simulink model "Plant"  (R2021a)
settings: Solver=VariableStepAuto  StartTime=0.0  StopTime=10.0  RelTol=1e-3
values from neighbouring files (symbols this model uses):
  bcx = 1e7    (= 10000000)    [Data.m]
  bcy = 1e8    (= 100000000)    [Data.m]
  bEh = 2*(bhd + bhm*ih^2)/rhd^2    (= 31004.4444444)    [Data.m]
  bEtd = (btd + btm*it^2)/rtd^2    (= 21607.2)    [Data.m]
  bhb = 1.0e8    (= 100000000)    [Data.m]
  bhEb = 2.2e9    (= 2200000000)    [Data.m]
  bt = 90    [Data.m]
  btb = 5.0e6    (= 5000000)    [Data.m]
  btw = 3e3    (= 3000)    [Data.m]
  bwu = 150    [Data.m]
  Container1_x0 = -15    [Data.m]
  Container1_y0 = 2.2    [Data.m]
  containerLayout = randi([0, maxContainers], 1, columns)    [Data.m]
  containerMasses = randi([Mc_range(1), Mc_range(2)], 1, columns)    [Data.m]
  dlh0 = 0    [Data.m]    (also in test__TLK.m; test_hoist.m; test_trolley.m)
  dxt0 = 0    [Data.m]    (also in test__TLK.m; test_hoist.m; test_trolley.m)
  dxtd0 = 0    [Data.m]    (also in test__TLK.m; test_hoist.m; test_trolley.m)
  g = 9.80665    [Data.m]
  Hc = 2.5    [Data.m]
  hoist_v115 = 115    [Data.m]
  ih = 22    [Data.m]
  it = 30    [Data.m]
  Kcy = 1.8e9    (= 1800000000)    [Data.m]
  Ktw = 4.8e5    (= 480000)    [Data.m]
  kwu = 2.36e8    (= 236000000)    [Data.m]
  lh0 = 10    [Data.m]    (also in test__TLK.m = 54.35; test_hoist.m = 20; test_trolley.m = 6)
  MAX_CABLE_LENGTH = y_axis(2) - y_axis(1)    [Data.m]
  Mc_range = [2000 50000]    [Data.m]
  MEh = 2*(Jhd_hEb + Jhm_hb * ih^2)/rhd^2    (= 65137.7777778)    [Data.m]
  MEtd = (Jtd + Jtm_tb*it^2)/rtd^2    (= 30000)    [Data.m]
  Ms = 15000    [Data.m]
  Mt = 30000    [Data.m]
  rhd = 0.75    [Data.m]
  rtd = 0.5    [Data.m]
  SHIP_LIMIT = x_axis(2)    [Data.m]
  SHORE_LIMIT = x_axis(1)    [Data.m]
  Thb_max = 5.0e4    (= 50000)    [Data.m]
  ThEb_max = 1.1e6    (= 1100000)    [Data.m]
  theta_hm0 = 0    [Data.m]    (also in test__TLK.m; test_hoist.m; test_trolley.m)
  theta_tm0 = 0    [Data.m]    (also in test__TLK.m; test_hoist.m; test_trolley.m)
  Ttb_max = 5.0e-3    (= 0.005)    [Data.m]
  Vlx0 = 0    [Data.m]    (also in test__TLK.m; test_hoist.m; test_trolley.m)
  Vly0 = 0    [Data.m]    (also in test__TLK.m; test_hoist.m; test_trolley.m)
  x_axis = [-30 50]    [Data.m]
  xl0 = xt0    (= 1)    [Data.m]    (also in test__TLK.m = 10.55; test_hoist.m = -20; test_trolley.m = -25)
  xt0 = 1    [Data.m]    (also in test__TLK.m = 10.55; test_hoist.m = -20; test_trolley.m = -25)
  xtd0 = xt0    (= 1)    [Data.m]    (also in test__TLK.m = 10.55; test_hoist.m = -20; test_trolley.m = -25)
  y_axis = [-20 40]    [Data.m]
  yl0 = Yt0 - lh0    (= 35)    [Data.m]    (also in test__TLK.m = Yt0 - lh0; test_hoist.m = Yt0 - lh0; test_trolley.m = Yt0 - lh0 - 1/4 * (Ms*g)/(kwu/(2*lh0+110)))
  Yt0 = 45    [Data.m]
libraries: simulink x3, vrlib x1
settings Model: Creator=jpss8  LastModifiedBy=ThnkPad

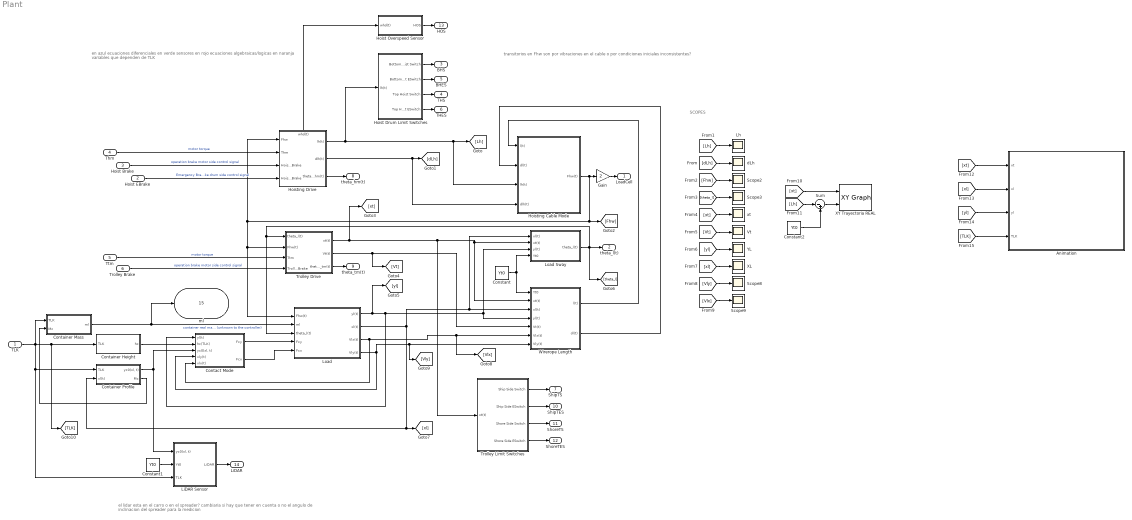
== system Plant ==
  note: SCOPES
  note: en azul ecuaciones diferenciales
      | en verde sensores
      | en rojo ecuaciones algebraicas/logicas
      | en naranja variables que dependen de TLK
  note: el lidar esta en el carro o en el spreader? cambiaria si hay que tener en cuenta o no el angulo de inclinacion del spreader para la medicion
  note: transitorios en Fhw son por vibraciones en el cable o por condiciones iniciales inconsistentes?
  TLK : Inport
  Hoist EBrake : Inport  Port=2
  Hoist Brake : Inport  Port=3
  Thm : Inport  Port=4
  Ttm : Inport  Port=5
  Trolley Brake : Inport  Port=6
  Animation : Subsystem
  Constant : Constant  Value=Yt0
  Constant1 : Constant  Value=Yt0
  Constant2 : Constant  Value=Yt0
  Contact Mode : Subsystem
  Container Height : Subsystem
  Container Mass : Subsystem
  Container Profile : Subsystem
  Gain : Gain  Gain=2
  Hoist Drum Limit Switches : Subsystem
  Hoist Overspeed Sensor : Subsystem
  Hoisting Cable Mode : Subsystem
  Hoisting Drive : Subsystem
      settings: PortSchema="{\"entries\":[{\"content\":{\"sides\":[{\"content\":{\"connectorIds\":[\"In1\",\"In2\",\"In3\",\"In4\"]},\"type\":\"ConnectorPlacement.EquallySpacedRectSide\",\"uuid\":\"6fd1770e-d7ed-4f51-91a0-0929c8efe1d3\"},{\"content\":{\"connectorIds\":[\"Out1\",\"Out2\",\"Out3\"],\"side\":\"RIGHT\"},\"type\":\"ConnectorPlacement.EquallySpacedRectSide\",\"uuid\":\"8b4207e8-a8fb-49cf-b187-d50d58bbe698\"},{\"content\":{\"connectorIds\":[\"Out4\"],\"side\":\"TOP\"},\"type\":\"ConnectorPlacement.EquallySpacedRectSide\",\"uuid\":\"5319a049-552f-4b27-a7d1-196eaf1861ff\"}]},\"type\":\"ConnectorPlacement.EquallySpacedConnector\",\"uuid\":\"15d51aa7-7d1b-46b1-a1b4-72147bb9bc95\"}],\"packageUris\":[\"http://schema.mathworks.com/mf0/Connector/R2020b\"],\"version\":\"1.0\"}"
  Lh : Scope
  LiDAR Sensor : Subsystem
  Load : Subsystem
  Load Sway : Subsystem
  Scope{2..3,8..9} (4 alike) : Scope
  Sum : Sum  Inputs=|-+
  Trolley Drive : Subsystem
  Trolley Limit Switches : Subsystem
  Vt : Scope
  Wirerope Length : Subsystem
  XL : Scope
  XY Trayectoria REAL : simulink/Sinks/XY Graph  xmin=x_axis(1)  xmax=x_axis(2)  ymin=y_axis(1)  ymax=y_axis(2)  st=-1
  YL : Scope
  dLh : Scope
  xt : Scope
  LoadCell : Outport
  theta_l(t) : Outport  Port=2
  BHS : Outport  Port=3
  THS : Outport  Port=4
  BHES : Outport  Port=5
  THES : Outport  Port=6
  ShipTS : Outport  Port=7
  theta_hm(t) : Outport  Port=8
  theta_tm(t) : Outport  Port=9
  ShipTES : Outport  Port=10
  ShoreTS : Outport  Port=11
  ShoreTES : Outport  Port=12
  HOS : Outport  Port=13
  LiDAR : Outport  Port=14
  ml : Outport  Port=15
  wires:
  Load/2(xl(t)) -> [xl], Container Profile/2(xl(t)), Load Sway/1(xl(t)), Wirerope Length/3(xl(t))
  Constant/1 -> Load Sway/4(Yt0), Wirerope Length/1(Yt0)
  Contact Mode/1(Fcy) -> Load/4(Fcy)
  Contact Mode/2(Fcx) -> Load/5(Fcx)
  Load/4(Vly(t)) -> Contact Mode/4(vly(t)), [Vly], Wirerope Length/7(Vly(t))
  Load/3(Vlx(t)) -> Contact Mode/5(vlx(t)), [Vlx], Wirerope Length/6(Vlx(t))
  Container Height/1(hc) -> Contact Mode/2(hc(TLK))
  Load Sway/1(theta_l(t)) -> [theta_l], theta_l(t)/1, Load/3(theta_l(t)), Trolley Drive/1(theta_l(t))
  Container Mass/1(ml) -> ml/1, Load/2(ml)  "container real mass (unknown to the controller)"
  Trolley Drive/1(xt(t)) -> [xt], Trolley Limit Switches/1(xt(t)), Wirerope Length/2(xt(t)), Load Sway/2(xt(t))
  Hoisting Drive/1(lh(t)) -> Hoist Drum Limit Switches/1(lh(t)), [Lh], Hoisting Cable Mode/3(lh(t))
  Hoisting Drive/2(dlh(t)) -> Hoisting Cable Mode/4(dlh(t)), [dLh]
  Wirerope Length/1(l(t)) -> Hoisting Cable Mode/1(l(t))
  Wirerope Length/2(dl(t)) -> Hoisting Cable Mode/2(dl(t))
  Hoisting Cable Mode/1(Fhw(t)) -> Gain/1, [Fhw], Load/1(Fhw(t)), Trolley Drive/2(Fhw(t)), Hoisting Drive/1(Fhw)
  Ttm/1 -> Trolley Drive/3(Ttm)  "motor torque"
  Thm/1 -> Hoisting Drive/2(Thm)  "motor torque"
  Trolley Brake/1 -> Trolley Drive/4(Trolley Brake)  "operation brake motor side control signal"
  Hoist Brake/1 -> Hoisting Drive/3(Hoist Brake)  "operation brake motor side control signal"
  Hoist EBrake/1 -> Hoisting Drive/4(Hoist EBrake)  "Emergency Brake drum side control signal"
  TLK/1 -> LiDAR Sensor/3(TLK), Container Profile/1(TLK), Container Mass/1(TLK), [TLK], Container Height/1(TLK)
  Hoisting Drive/3(theta_hm(t)) -> theta_hm(t)/1
  Trolley Drive/3(theta_tm(t)) -> theta_tm(t)/1
  Hoist Drum Limit Switches/1(Bottom Hoist Switch) -> BHS/1
  Hoist Drum Limit Switches/3(Top Hoist Switch) -> THS/1
  Hoist Drum Limit Switches/2(Bottom Hoist ESwitch) -> BHES/1
  Hoist Drum Limit Switches/4(Top Hoist ESwitch) -> THES/1
  Trolley Limit Switches/1(Ship Side Switch) -> ShipTS/1
  Trolley Limit Switches/2(Ship Side ESwitch) -> ShipTES/1
  Trolley Limit Switches/3(Shore Side Switch) -> ShoreTS/1
  Trolley Limit Switches/4(Shore Side ESwitch) -> ShoreTES/1
  Container Profile/1("yc0(xl, t)") -> LiDAR Sensor/1("yc0(xl, t)"), Contact Mode/3("yc0(xl, t)")
  Gain/1 -> LoadCell/1
  Hoisting Drive/4(whd(t)) -> Hoist Overspeed Sensor/1(whd(t))
  Hoist Overspeed Sensor/1(HOS) -> HOS/1
  Trolley Drive/2(Vt(t)) -> [Vt], Wirerope Length/5(Vt(t))
  LiDAR Sensor/1(LiDAR) -> LiDAR/1
  Load/1(yl(t)) -> [yl], Contact Mode/1(yl(t)), Load Sway/3(yl(t)), Wirerope Length/4(yl(t))
  Constant1/1 -> LiDAR Sensor/2(Yt0)
  [Vlx] -> Scope9/1
  [Vly] -> Scope8/1
  [xl] -> XL/1
  [yl] -> YL/1
  [Vt] -> Vt/1
  [xt] -> xt/1
  [theta_l] -> Scope3/1
  [Fhw] -> Scope2/1
  [dLh] -> dLh/1
  [Lh] -> Lh/1
  Container Profile/2(Mc) -> Container Mass/2(Mc)
  [xt] -> XY Trayectoria REAL/1
  Sum/1 -> XY Trayectoria REAL/2
  [Lh] -> Sum/1
  Constant2/1 -> Sum/2
  [xt] -> Animation/1(xt)
  [xl] -> Animation/2(xl)
  [yl] -> Animation/3(yl)
  [TLK] -> Animation/4(TLK)

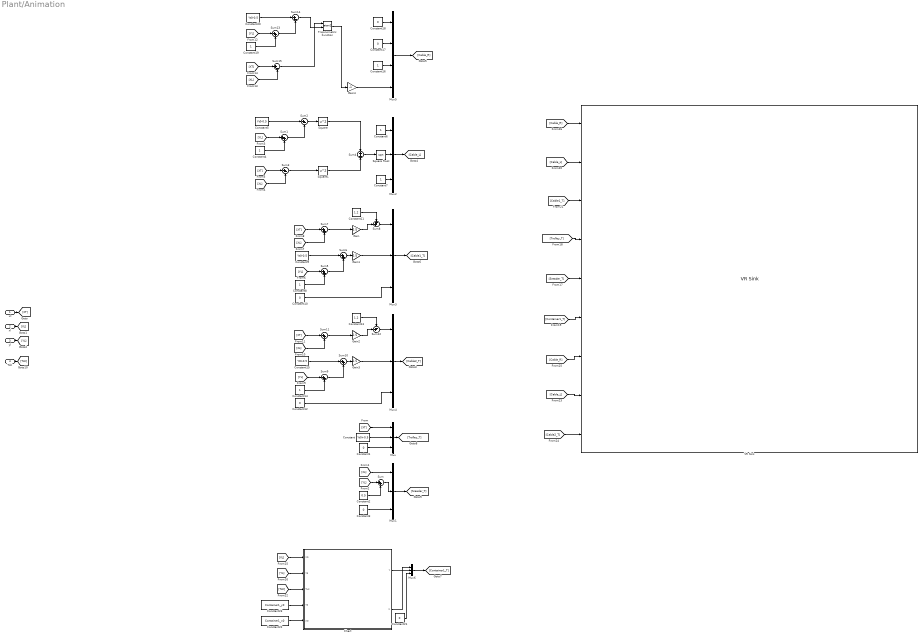
== system Plant/Animation ==
  xt : Inport
  xl : Inport  Port=2
  yl : Inport  Port=3
  TLK : Inport  Port=4
  Chart : Stateflow chart  TreatAsAtomicUnit=on
  Constant : Constant  Value=Yt0+0.5
  Constant{1,3,10,12,17..18,21} (7 alike) : Constant  Value=0
  Constant11 : Constant  Value=1.2
  Constant13 : Constant  Value=1.2
  Constant{4,6..8,14,16,19} (7 alike) : Constant
  Constant{5,9,15,20} (4 alike) : Constant  Value=Yt0-0.5
  Constant2 : Constant  Value=0.5
  Constant22 : Constant  Value=Container1_x0
  Constant23 : Constant  Value=Container1_y0
  Gain{,1..3} (4 alike) : Gain  Gain=0.5
  Gain4 : Gain  Gain=-1
  Mux{,1..4,6} (6 alike) : Mux  Inputs=3
  Mux5 : Mux
  Square : Math  Operator=square  SaturateOnIntegerOverflow=on
  Square Root : Sqrt  SaturateOnIntegerOverflow=on
  Square1 : Math  Operator=square  SaturateOnIntegerOverflow=on
  Sum{,1,5..7,9..11,13} (9 alike) : Sum  Inputs=|++
  Sum12 : Sum  Inputs=-+|
  Sum{2..3,14..15} (4 alike) : Sum  Inputs=|+-
  Sum4 : Sum
  Sum8 : Sum  Inputs=++|
  Trigonometric Function : Trigonometry  Operator=atan2
  VR Sink : vrlib/VR Sink  InstantiateOnLoad=on  SampleTime=0.1  ViewEnable=on  RemoteChange=off  RemoteView=off  FieldsWritten=cable1.rotation.4.1.1.double#cable1.scale.3.1.1.double#cable1.translation.3.1.1.double#Trolley.translation.3.1.1.double#Spreader.translation.3.1.1.double#ActiveContainer1.translation.3.1.1.double#cable2.rotation.4.1.1.double#cable2.scale.3.1.1.double#cable2.translation.3.1.1.double  WorldFileName=Animation.x3d  AutoView=off  VideoDimensions=[]  AllowVariableSize=off  FigureProperties="{'Position', 'Name', 'Viewpoint', 'CameraBound', 'CameraDirection', 'CameraPosition', 'CameraUpVector', 'ZoomFactor', 'Antialiasing', 'Headlight', 'Lighting', 'NavPanel', 'Sound', 'StatusBar', 'Stereo3D', 'Stereo3DCameraOffset', 'Stereo3DHIT', 'ToolBar', 'Textures', 'Transparency', 'Triad', 'Wireframe', 'NavZones', 'NavMode', 'NavSpeed', 'CaptureFileFormat', 'CaptureFileName', 'Record2DCompressMethod', 'Record2DCompressQuality', 'Record2D', 'Record2DFileName', 'Record2DFPS'; [1.0000000000000000e+00   7.6000000000000000e+01   1.3660000000000000e+03   6.4100000000000000e+02], '', '', 'on', [1.2372845022256038e-01   0.0000000000000000e+00  -9.9231611425267274e-01], [-2.0372126446111569e+01   2.5367790222167969e+01   1.7338674991649961e+02], [0.0000000000000000e+00   1.0000000000000000e+00   0.0000000000000000e+00], [1.0000000000000000e+00], 'on', 'on', 'on', 'halfbar', 'on', 'on', 'off', [1.0000000149011612e-01], [0.0000000000000000e+00], 'on', 'on', 'on', 'none', 'off', 'off', 'fly', 'normal', 'tif', '%f_anim_%n.tif', 'auto', [7.5000000000000000e+01], 'on', '%f_anim_%n.avi', 'auto'}"
  wires:
  Constant/1 -> Mux/2
  Constant1/1 -> Mux/3
  Constant3/1 -> Mux1/3
  Sum/1 -> Mux1/2
  Constant2/1 -> Sum/2
  xt/1 -> [XT]
  xl/1 -> [XL]
  yl/1 -> [YL]
  [XT] -> Mux/1
  [XL] -> Mux1/1
  [YL] -> Sum/1
  [YL] -> Sum1/1
  Constant4/1 -> Sum1/2
  Constant5/1 -> Sum2/1
  Sum1/1 -> Sum2/2
  Sum2/1 -> Square/1
  Sum3/1 -> Square1/1
  [XL] -> Sum3/2
  [XT] -> Sum3/1
  Square/1 -> Sum4/1
  Square1/1 -> Sum4/2
  Sum4/1 -> Square Root/1
  Square Root/1 -> Mux2/2
  Constant7/1 -> Mux2/3
  Constant6/1 -> Mux2/1
  Constant9/1 -> Sum6/1
  [YL] -> Sum5/1
  Constant8/1 -> Sum5/2
  Sum5/1 -> Sum6/2
  [XT] -> Sum7/1
  [XL] -> Sum7/2
  Sum7/1 -> Gain/1
  Sum6/1 -> Gain1/1
  Gain1/1 -> Mux3/2
  Constant10/1 -> Mux3/3
  Sum8/1 -> Mux3/1
  Gain/1 -> Sum8/2
  Constant11/1 -> Sum8/1
  Sum10/1 -> Gain3/1
  Gain2/1 -> Sum12/2
  Constant14/1 -> Sum9/2
  [YL] -> Sum9/1
  Sum9/1 -> Sum10/2
  Constant12/1 -> Mux4/3
  [XT] -> Sum11/1
  Constant13/1 -> Sum12/1
  Gain3/1 -> Mux4/2
  Sum12/1 -> Mux4/1
  Constant15/1 -> Sum10/1
  Sum11/1 -> Gain2/1
  [XL] -> Sum11/2
  Constant17/1 -> Mux5/2
  Constant16/1 -> Mux5/3
  Constant18/1 -> Mux5/1
  Sum14/1 -> Trigonometric Function/2
  Constant20/1 -> Sum14/1
  [XT] -> Sum15/1
  [YL] -> Sum13/1
  [XL] -> Sum15/2
  Constant19/1 -> Sum13/2
  Sum13/1 -> Sum14/2
  Sum15/1 -> Trigonometric Function/1
  Trigonometric Function/1 -> Gain4/1
  Gain4/1 -> Mux5/4
  Chart/2(X) -> Mux6/1
  Constant21/1 -> Mux6/3
  Chart/1(Y) -> Mux6/2
  Mux4/1 -> [Cable2_T]
  Mux2/1 -> [Cable_L]
  Mux5/1 -> [Cable_R]
  Mux3/1 -> [Cable1_T]
  Mux6/1 -> [Container1_T]
  Mux1/1 -> [Sreader_T]
  Mux/1 -> [Trolley_T]
  [XL] -> Chart/1(XS)
  [YL] -> Chart/2(YS)
  TLK/1 -> [TLK]
  [TLK] -> Chart/3(TLK)
  Constant23/1 -> Chart/4(Y0)
  Constant22/1 -> Chart/5(X0)
  [Cable_R] -> VR Sink/1
  [Cable_L] -> VR Sink/2
  [Cable1_T] -> VR Sink/3
  [Trolley_T] -> VR Sink/4
  [Sreader_T] -> VR Sink/5
  [Container1_T] -> VR Sink/6
  [Cable_R] -> VR Sink/7
  [Cable_L] -> VR Sink/8
  [Cable2_T] -> VR Sink/9

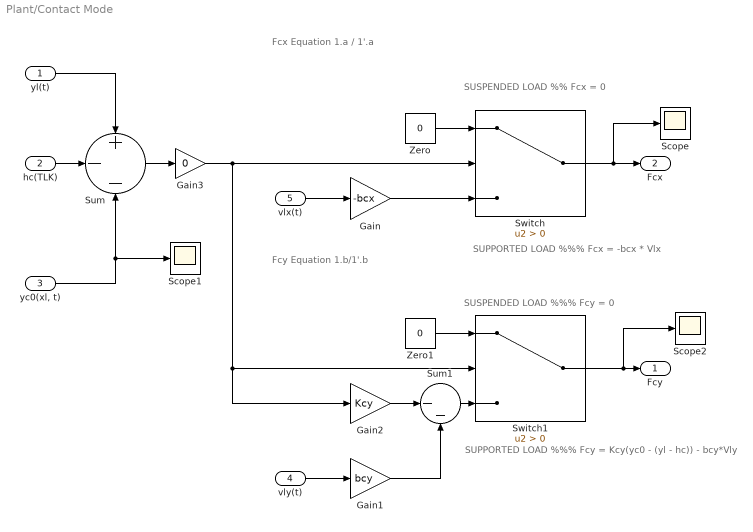
== system Plant/Contact Mode ==
  note: Fcy Equation 1.b/1'.b
  note: Fcx Equation 1.a / 1'.a
  note: SUPPORTED LOAD %%% Fcx = -bcx * Vlx
  note: SUSPENDED LOAD %% Fcx = 0
  note: SUSPENDED LOAD %%% Fcy = 0
  note: SUPPORTED LOAD %%% Fcy = Kcy(yc0 - (yl - hc)) - bcy*Vly
  yl(t) : Inport
  hc(TLK) : Inport  Port=2
  "yc0(xl, t)" : Inport  Port=3
  vly(t) : Inport  Port=4
  vlx(t) : Inport  Port=5
  Gain : Gain  Gain=-bcx
  Gain1 : Gain  Gain=bcy
  Gain2 : Gain  Gain=Kcy
  Gain3 : Gain  Gain=0
  Scope : Scope
  Scope1 : Scope
  Scope2 : Scope
  Sum : Sum  Inputs=+--
  Sum1 : Sum  Inputs=|--
  Switch : Switch  Criteria=u2 > Threshold
  Switch1 : Switch  Criteria=u2 > Threshold
  Zero : Constant  Value=0  OutDataTypeStr=Inherit: Inherit via back propagation
  Zero1 : Constant  Value=0  OutDataTypeStr=Inherit: Inherit via back propagation
  Fcy : Outport
  Fcx : Outport  Port=2
  wires:
  yl(t)/1 -> Sum/1
  hc(TLK)/1 -> Sum/2
  Sum/1 -> Gain3/1
  Zero/1 -> Switch/1
  Switch/1 -> Scope/1, Fcx/1
  Zero1/1 -> Switch1/1
  Switch1/1 -> Scope2/1, Fcy/1
  Gain/1 -> Switch/3
  vlx(t)/1 -> Gain/1
  vly(t)/1 -> Gain1/1
  Sum1/1 -> Switch1/3
  Gain1/1 -> Sum1/2
  Gain2/1 -> Sum1/1
  "yc0(xl, t)"/1 -> Scope1/1, Sum/3
  Gain3/1 -> Switch/2, Gain2/1, Switch1/2

== system Plant/Container Height ==
  TLK : Inport
  Constant : Constant  Value=Hc
  Product : Product
  hc : Outport
  wires:
  TLK/1 -> Product/1  "Twist Locks Signal"
  Product/1 -> hc/1
  Constant/1 -> Product/2

== system Plant/Container Mass ==
  TLK : Inport
  Mc : Inport  Port=2
  Constant : Constant  Value=Ms
  Product : Product
  Sum : Sum  Inputs=|++
  ml : Outport
  wires:
  TLK/1 -> Product/1
  Constant/1 -> Sum/1
  Sum/1 -> ml/1
  Product/1 -> Sum/2
  Mc/1 -> Product/2

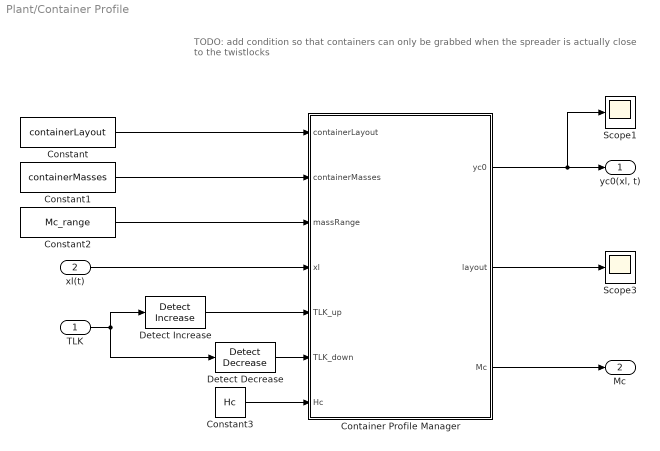
== system Plant/Container Profile ==
  note: TODO: add condition so that containers can only be grabbed when the spreader is actually close to the twistlocks
  TLK : Inport
  xl(t) : Inport  Port=2
  Constant : Constant  Value=containerLayout
  Constant1 : Constant  Value=containerMasses
  Constant2 : Constant  Value=Mc_range
  Constant3 : Constant  Value=Hc
  Container Profile Manager : Stateflow chart  TreatAsAtomicUnit=on
      settings: PortSchema="{\"entries\":[{\"content\":{\"sides\":[{\"content\":{\"connectorIds\":[\"In1\",\"In6\",\"In7\",\"In2\",\"In3\",\"In5\",\"In4\"]},\"type\":\"ConnectorPlacement.EquallySpacedRectSide\",\"uuid\":\"5766d641-49f2-4d27-af07-326f142e6aed\"},{\"content\":{\"connectorIds\":[\"Out1\",\"Out2\",\"Out3\"],\"side\":\"RIGHT\"},\"type\":\"ConnectorPlacement.EquallySpacedRectSide\",\"uuid\":\"189da8a7-e781-479b-88d0-249e58f15313\"},{\"content\":{\"connectorIds\":[],\"side\":\"TOP\"},\"type\":\"ConnectorPlacement.EquallySpacedRectSide\",\"uuid\":\"2ddba87e-7b61-4748-b795-d214d19f6f2a\"}]},\"type\":\"ConnectorPlacement.EquallySpacedConnector\",\"uuid\":\"5bdf3cb8-46a3-4ebe-84f7-15990506ca0e\"}],\"packageUris\":[\"http://schema.mathworks.com/mf0/Connector/R2020b\"],\"version\":\"1.0\"}"
  Detect Decrease : simulink/Logic and Bit Operations/Detect Decrease  vinit=0.0  OutDataTypeStr=boolean
  Detect Increase : simulink/Logic and Bit Operations/Detect Increase  vinit=0.0  OutDataTypeStr=boolean
  Scope1 : Scope
  Scope3 : Scope
  "yc0(xl, t)" : Outport
  Mc : Outport  Port=2
  wires:
  xl(t)/1 -> Container Profile Manager/2(xl)
  Constant3/1 -> Container Profile Manager/4(Hc)
  Detect Decrease/1 -> Container Profile Manager/5(TLK_down)
  Detect Increase/1 -> Container Profile Manager/3(TLK_up)
  Container Profile Manager/1(yc0) -> Scope1/1, "yc0(xl, t)"/1
  Constant/1 -> Container Profile Manager/1(containerLayout)
  TLK/1 -> Detect Increase/1, Detect Decrease/1
  Container Profile Manager/2(layout) -> Scope3/1
  Constant1/1 -> Container Profile Manager/6(containerMasses)
  Constant2/1 -> Container Profile Manager/7(massRange)
  Container Profile Manager/3(Mc) -> Mc/1

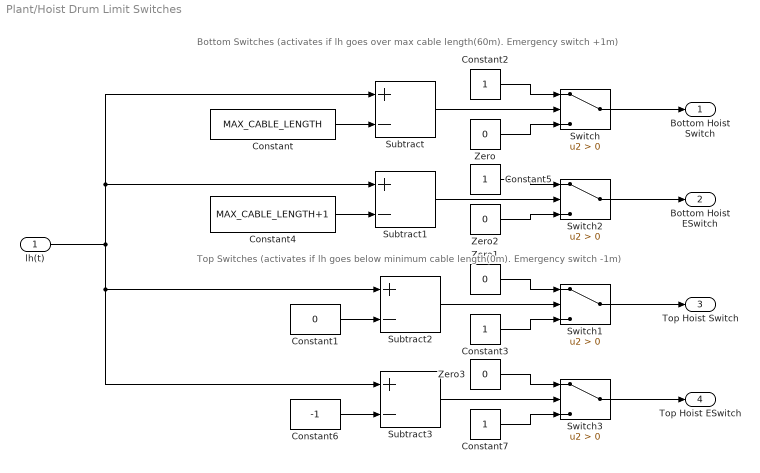
== system Plant/Hoist Drum Limit Switches ==
  note: Top Switches (activates if lh goes below minimum cable length(0m). Emergency switch -1m)
  note: Bottom Switches (activates if lh goes over max cable length(60m). Emergency switch +1m)
  lh(t) : Inport
  Constant : Constant  Value=MAX_CABLE_LENGTH
  Constant1 : Constant  Value=0
  Constant{2..3,5,7} (4 alike) : Constant
  Constant4 : Constant  Value=MAX_CABLE_LENGTH+1
  Constant6 : Constant  Value=-1
  Subtract{,1..3} (4 alike) : Sum  Inputs=+-
  Switch{,1..3} (4 alike) : Switch  Criteria=u2 > Threshold
  Zero{,1..3} (4 alike) : Constant  Value=0  OutDataTypeStr=Inherit: Inherit via back propagation
  Bottom Hoist Switch : Outport
  Bottom Hoist ESwitch : Outport  Port=2
  Top Hoist Switch : Outport  Port=3
  Top Hoist ESwitch : Outport  Port=4
  wires:
  Constant/1 -> Subtract/2
  Constant1/1 -> Subtract2/2
  Subtract/1 -> Switch/2
  Switch1/1 -> Top Hoist Switch/1
  Switch/1 -> Bottom Hoist Switch/1
  Subtract2/1 -> Switch1/2
  Zero1/1 -> Switch1/1
  Constant3/1 -> Switch1/3
  Zero/1 -> Switch/3
  Constant2/1 -> Switch/1
  Constant4/1 -> Subtract1/2
  Constant5/1 -> Switch2/1
  Zero2/1 -> Switch2/3
  Switch2/1 -> Bottom Hoist ESwitch/1
  Subtract1/1 -> Switch2/2
  Constant7/1 -> Switch3/3
  Zero3/1 -> Switch3/1
  Subtract3/1 -> Switch3/2
  Switch3/1 -> Top Hoist ESwitch/1
  Constant6/1 -> Subtract3/2
  lh(t)/1 -> Subtract1/1, Subtract/1, Subtract2/1, Subtract3/1

== system Plant/Hoist Overspeed Sensor ==
  whd(t) : Inport
  Constant : Constant
  Constant1 : Constant  Value=hoist_v115
  Sum : Sum  Inputs=|+-
  Switch : Switch  Criteria=u2 > Threshold
  Zero : Constant  Value=0  OutDataTypeStr=Inherit: Inherit via back propagation
  HOS : Outport
  wires:
  whd(t)/1 -> Sum/1
  Switch/1 -> HOS/1
  Zero/1 -> Switch/3
  Constant/1 -> Switch/1
  Constant1/1 -> Sum/2
  Sum/1 -> Switch/2

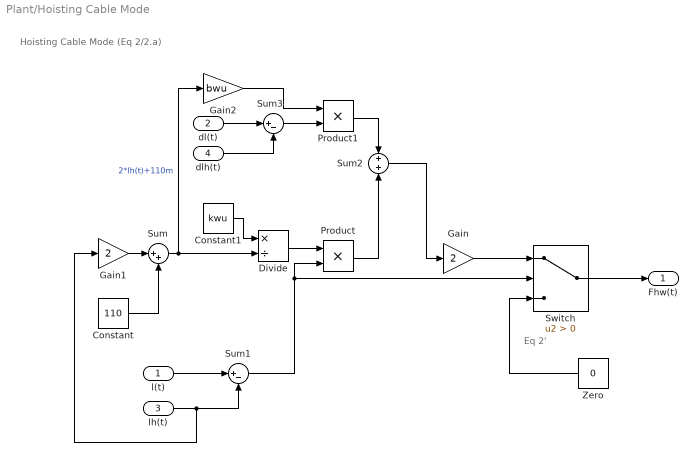
== system Plant/Hoisting Cable Mode ==
  note: Eq 2'
  note: Hoisting Cable Mode (Eq 2/2.a)
  l(t) : Inport
  dl(t) : Inport  Port=2
  lh(t) : Inport  Port=3
  dlh(t) : Inport  Port=4
  Constant : Constant  Value=110
  Constant1 : Constant  Value=kwu
  Divide : Product  Inputs=*/
  Gain : Gain  Gain=2
  Gain1 : Gain  Gain=2
  Gain2 : Gain  Gain=bwu
  Product : Product
  Product1 : Product
  Sum : Sum  Inputs=|++
  Sum1 : Sum  Inputs=|+-
  Sum2 : Sum  Inputs=+|+
  Sum3 : Sum  Inputs=|+-
  Switch : Switch  Criteria=u2 > Threshold
  Zero : Constant  Value=0  OutDataTypeStr=Inherit: Inherit via back propagation
  Fhw(t) : Outport
  wires:
  lh(t)/1 -> Sum1/2, Gain1/1
  l(t)/1 -> Sum1/1
  Switch/1 -> Fhw(t)/1
  Zero/1 -> Switch/3
  dlh(t)/1 -> Sum3/2
  Sum3/1 -> Product1/2
  Gain1/1 -> Sum/1
  Constant/1 -> Sum/2
  Constant1/1 -> Divide/1
  Sum/1 -> Gain2/1, Divide/2  "2*lh(t)+110m"
  Divide/1 -> Product/1
  Gain/1 -> Switch/1
  Product1/1 -> Sum2/1
  Product/1 -> Sum2/2
  Sum2/1 -> Gain/1
  Gain2/1 -> Product1/1
  dl(t)/1 -> Sum3/1
  Sum1/1 -> Product/2, Switch/2

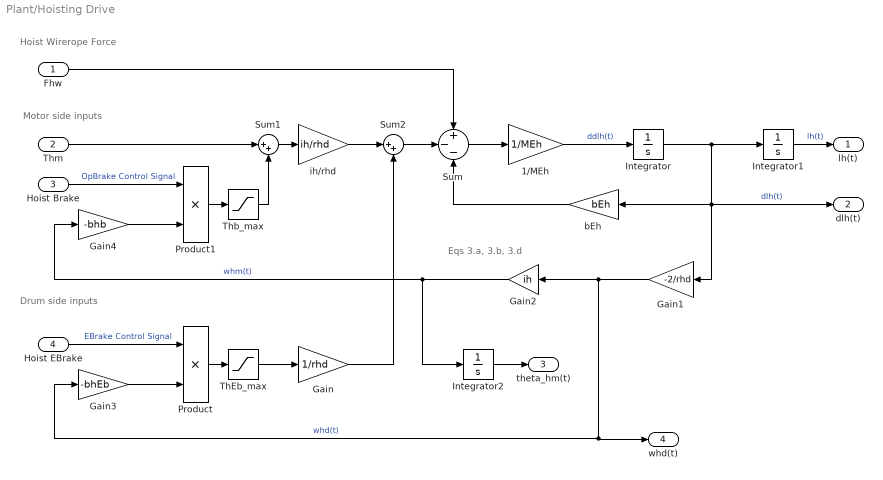
== system Plant/Hoisting Drive ==
  note: Eqs 3.a, 3.b, 3.d
  note: Hoist Wirerope Force
  note: Drum side inputs
  note: Motor side inputs
  Fhw : Inport
  Thm : Inport  Port=2
  Hoist Brake : Inport  Port=3
  Hoist EBrake : Inport  Port=4
  1/MEh : Gain  Gain=1/MEh
  Gain : Gain  Gain=1/rhd
  Gain1 : Gain  Gain=-2/rhd
  Gain2 : Gain  Gain=ih
  Gain3 : Gain  Gain=-bhEb
  Gain4 : Gain  Gain=-bhb
  Integrator : Integrator  InitialCondition=dlh0
  Integrator1 : Integrator  InitialCondition=lh0
  Integrator2 : Integrator  InitialCondition=theta_hm0
  Product : Product
  Product1 : Product
  Sum : Sum  Inputs=+--
  Sum1 : Sum  Inputs=|++
  Sum2 : Sum  Inputs=|++
  ThEb_max : Saturate  UpperLimit=ThEb_max  LowerLimit=-ThEb_max
  Thb_max : Saturate  UpperLimit=Thb_max  LowerLimit=-Thb_max
  bEh : Gain  Gain=bEh
  ih/rhd : Gain  Gain=ih/rhd
  lh(t) : Outport
  dlh(t) : Outport  Port=2
  theta_hm(t) : Outport  Port=3
  whd(t) : Outport  Port=4
  wires:
  Integrator/1 -> Integrator1/1, bEh/1, Gain1/1, dlh(t)/1  "dlh(t)"
  bEh/1 -> Sum/3
  Sum/1 -> 1/MEh/1
  Fhw/1 -> Sum/1
  1/MEh/1 -> Integrator/1  "ddlh(t)"
  Sum1/1 -> ih/rhd/1
  Thm/1 -> Sum1/1
  Gain/1 -> Sum2/2
  ih/rhd/1 -> Sum2/1
  Sum2/1 -> Sum/2
  Gain1/1 -> whd(t)/1, Gain3/1, Gain2/1  "whd(t)"
  Gain2/1 -> Integrator2/1, Gain4/1  "whm(t)"
  Hoist EBrake/1 -> Product/1  "EBrake Control Signal"
  Product/1 -> ThEb_max/1
  Gain3/1 -> Product/2
  ThEb_max/1 -> Gain/1
  Product1/1 -> Thb_max/1
  Hoist Brake/1 -> Product1/1  "OpBrake Control Signal"
  Thb_max/1 -> Sum1/2
  Gain4/1 -> Product1/2
  Integrator2/1 -> theta_hm(t)/1
  Integrator1/1 -> lh(t)/1  "lh(t)"

== system Plant/LiDAR Sensor ==
  "yc0(xl, t)" : Inport
  Yt0 : Inport  Port=2
  TLK : Inport  Port=3
  NOT : Logic  Operator=NOT  IconShape=distinctive  AllPortsSameDT=off  OutDataTypeStr=boolean
  Product : Product
  Sum : Sum  Inputs=|+-
  LiDAR : Outport
  wires:
  Yt0/1 -> Sum/1
  "yc0(xl, t)"/1 -> Sum/2
  Product/1 -> LiDAR/1
  Sum/1 -> Product/1
  TLK/1 -> NOT/1
  NOT/1 -> Product/2

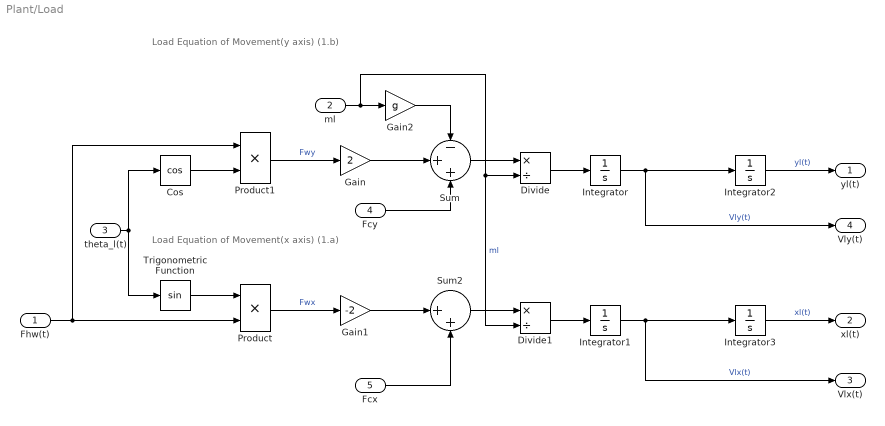
== system Plant/Load ==
  note: Load Equation of Movement(x axis) (1.a)
  note: Load Equation of Movement(y axis) (1.b)
  Fhw(t) : Inport
  ml : Inport  Port=2
  theta_l(t) : Inport  Port=3
  Fcy : Inport  Port=4
  Fcx : Inport  Port=5
  Cos : Trigonometry  Operator=cos
  Divide : Product  Inputs=*/
  Divide1 : Product  Inputs=*/
  Gain : Gain  Gain=2
  Gain1 : Gain  Gain=-2
  Gain2 : Gain  Gain=g
  Integrator : Integrator  InitialCondition=Vly0
  Integrator1 : Integrator  InitialCondition=Vlx0
  Integrator2 : Integrator  InitialCondition=yl0
  Integrator3 : Integrator  InitialCondition=xl0
  Product : Product
  Product1 : Product
  Sum : Sum  Inputs=-++
  Sum2 : Sum  Inputs=|++
  Trigonometric Function : Trigonometry
  yl(t) : Outport
  xl(t) : Outport  Port=2
  Vlx(t) : Outport  Port=3
  Vly(t) : Outport  Port=4
  wires:
  Fhw(t)/1 -> Product/2, Product1/1
  Trigonometric Function/1 -> Product/1
  Cos/1 -> Product1/2
  Product/1 -> Gain1/1  "Fwx"
  Product1/1 -> Gain/1  "Fwy"
  theta_l(t)/1 -> Trigonometric Function/1, Cos/1
  Gain/1 -> Sum/2
  Fcy/1 -> Sum/3
  Gain1/1 -> Sum2/1
  Fcx/1 -> Sum2/2
  Sum/1 -> Divide/1
  Gain2/1 -> Sum/1
  ml/1 -> Gain2/1, Divide1/2, Divide/2  "ml"
  Sum2/1 -> Divide1/1
  Divide/1 -> Integrator/1
  Divide1/1 -> Integrator1/1
  Integrator/1 -> Integrator2/1, Vly(t)/1  "Vly(t)"
  Integrator1/1 -> Integrator3/1, Vlx(t)/1  "Vlx(t)"
  Integrator2/1 -> yl(t)/1  "yl(t)"
  Integrator3/1 -> xl(t)/1  "xl(t)"

== system Plant/Load Sway ==
  note: Load Sway Angle (Eq 0.d)
  xl(t) : Inport
  xt(t) : Inport  Port=2
  yl(t) : Inport  Port=3
  Yt0 : Inport  Port=4
  Atan2 : Trigonometry  Operator=atan2
  Sum : Sum  Inputs=+-
  Sum1 : Sum  Inputs=+-
  theta_l(t) : Outport
  wires:
  Yt0/1 -> Sum/1
  yl(t)/1 -> Sum/2
  xl(t)/1 -> Sum1/1
  xt(t)/1 -> Sum1/2
  Sum1/1 -> Atan2/1  "xl-xt"
  Sum/1 -> Atan2/2  "yl-yt"
  Atan2/1 -> theta_l(t)/1

== system Plant/Trolley Drive ==
  theta_l(t) : Inport
  Fhw(t) : Inport  Port=2
  Ttm : Inport  Port=3
  Trolley Brake : Inport  Port=4
  Drum Subsystem : Subsystem
  Trolley Cable Mode : Subsystem
  Trolley Subsystem : Subsystem
  xt(t) : Outport
  Vt(t) : Outport  Port=2
  theta_tm(t) : Outport  Port=3
  wires:
  theta_l(t)/1 -> Trolley Subsystem/1(theta_l(t))
  Fhw(t)/1 -> Trolley Subsystem/2(Fhw(t))
  Ttm/1 -> Drum Subsystem/2(Ttm)
  Trolley Subsystem/1(xt(t)) -> Trolley Cable Mode/1(xt(t)), xt(t)/1
  Trolley Subsystem/2(dxt(t)) -> Vt(t)/1, Trolley Cable Mode/2(dxt(t))
  Drum Subsystem/1(xtd(t)) -> Trolley Cable Mode/3(xtd(t))
  Drum Subsystem/2(dxtd(t)) -> Trolley Cable Mode/4(dxtd(t))
  Trolley Cable Mode/1(Ftw) -> [A]  "Ftw"
  [A] -> Trolley Subsystem/3(Ftw(t)), Drum Subsystem/1(Ftw(t))
  Trolley Brake/1 -> Drum Subsystem/3(Ttb)  "OpBrake Control Signal"
  Drum Subsystem/3(theta_tm(t)) -> theta_tm(t)/1

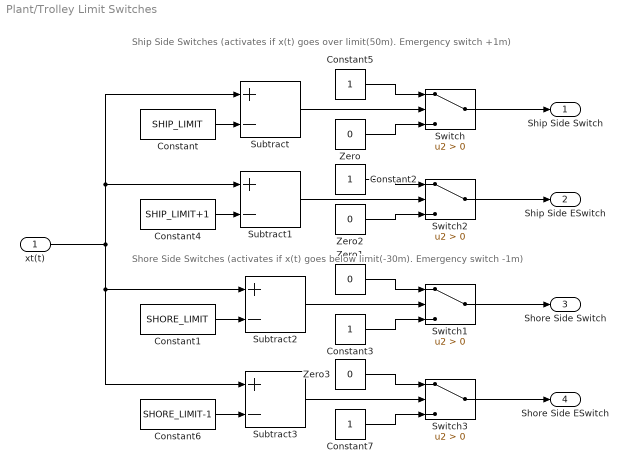
== system Plant/Trolley Limit Switches ==
  note: Ship Side Switches (activates if x(t) goes over limit(50m). Emergency switch +1m)
  note: Shore Side Switches (activates if x(t) goes below limit(-30m). Emergency switch -1m)
  xt(t) : Inport
  Constant : Constant  Value=SHIP_LIMIT
  Constant1 : Constant  Value=SHORE_LIMIT
  Constant{2..3,5,7} (4 alike) : Constant
  Constant4 : Constant  Value=SHIP_LIMIT+1
  Constant6 : Constant  Value=SHORE_LIMIT-1
  Subtract{,1..3} (4 alike) : Sum  Inputs=+-
  Switch{,1..3} (4 alike) : Switch  Criteria=u2 > Threshold
  Zero{,1..3} (4 alike) : Constant  Value=0  OutDataTypeStr=Inherit: Inherit via back propagation
  Ship Side Switch : Outport
  Ship Side ESwitch : Outport  Port=2
  Shore Side Switch : Outport  Port=3
  Shore Side ESwitch : Outport  Port=4
  wires:
  Zero1/1 -> Switch1/1
  Constant4/1 -> Subtract1/2
  Constant5/1 -> Switch/1
  Constant/1 -> Subtract/2
  Switch/1 -> Ship Side Switch/1
  Zero/1 -> Switch/3
  Constant6/1 -> Subtract3/2
  Switch3/1 -> Shore Side ESwitch/1
  Switch1/1 -> Shore Side Switch/1
  Constant7/1 -> Switch3/3
  Zero3/1 -> Switch3/1
  Constant1/1 -> Subtract2/2
  Subtract2/1 -> Switch1/2
  xt(t)/1 -> Subtract2/1, Subtract3/1, Subtract1/1, Subtract/1
  Subtract/1 -> Switch/2
  Zero2/1 -> Switch2/3
  Constant2/1 -> Switch2/1
  Subtract3/1 -> Switch3/2
  Constant3/1 -> Switch1/3
  Switch2/1 -> Ship Side ESwitch/1
  Subtract1/1 -> Switch2/2

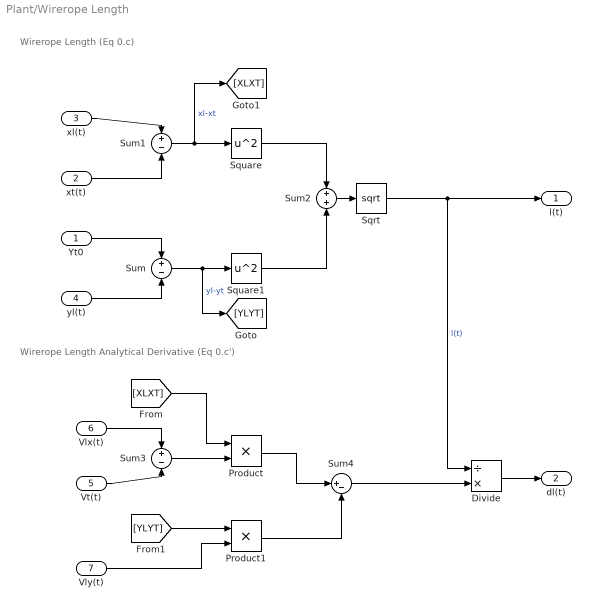
== system Plant/Wirerope Length ==
  note: Wirerope Length Analytical Derivative (Eq 0.c')
  note: Wirerope Length (Eq 0.c)
  Yt0 : Inport
  xt(t) : Inport  Port=2
  xl(t) : Inport  Port=3
  yl(t) : Inport  Port=4
  Vt(t) : Inport  Port=5
  Vlx(t) : Inport  Port=6
  Vly(t) : Inport  Port=7
  Divide : Product  Inputs=/*
  Product : Product
  Product1 : Product
  Sqrt : Sqrt  SaturateOnIntegerOverflow=on
  Square : Math  Operator=square  SaturateOnIntegerOverflow=on
  Square1 : Math  Operator=square  SaturateOnIntegerOverflow=on
  Sum : Sum  Inputs=+-
  Sum1 : Sum  Inputs=+-
  Sum2 : Sum
  Sum3 : Sum  Inputs=+-
  Sum4 : Sum  Inputs=|+-
  l(t) : Outport
  dl(t) : Outport  Port=2
  wires:
  Yt0/1 -> Sum/1
  yl(t)/1 -> Sum/2
  xl(t)/1 -> Sum1/1
  xt(t)/1 -> Sum1/2
  Sqrt/1 -> Divide/1, l(t)/1  "l(t)"
  Sum1/1 -> [XLXT], Square/1  "xl-xt"
  Sum/1 -> Square1/1, [YLYT]  "yl-yt"
  Square/1 -> Sum2/1
  Square1/1 -> Sum2/2
  Sum2/1 -> Sqrt/1
  Divide/1 -> dl(t)/1
  Vlx(t)/1 -> Sum3/1
  Vt(t)/1 -> Sum3/2
  Sum3/1 -> Product/2
  Product/1 -> Sum4/1
  Vly(t)/1 -> Product1/2
  Product1/1 -> Sum4/2
  Sum4/1 -> Divide/2
  [XLXT] -> Product/1
  [YLYT] -> Product1/1

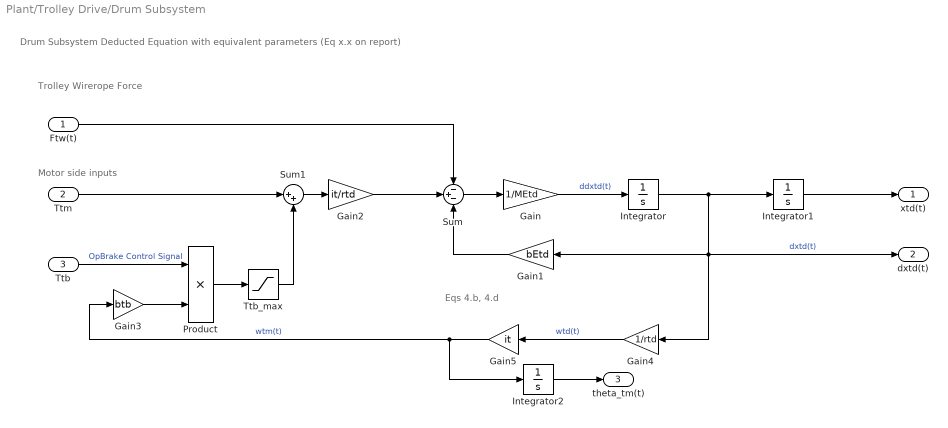
== system Plant/Trolley Drive/Drum Subsystem ==
  note: Eqs 4.b, 4.d
  note: Drum Subsystem Deducted Equation with equivalent parameters (Eq x.x on report)
  note: Trolley Wirerope Force
  note: Motor side inputs
  Ftw(t) : Inport
  Ttm : Inport  Port=2
  Ttb : Inport  Port=3
  Gain : Gain  Gain=1/MEtd
  Gain1 : Gain  Gain=bEtd
  Gain2 : Gain  Gain=it/rtd
  Gain3 : Gain  Gain=btb
  Gain4 : Gain  Gain=1/rtd
  Gain5 : Gain  Gain=it
  Integrator : Integrator  InitialCondition=dxtd0
  Integrator1 : Integrator  InitialCondition=xtd0
  Integrator2 : Integrator  InitialCondition=theta_tm0
  Product : Product
  Sum : Sum  Inputs=-+-
  Sum1 : Sum  Inputs=|++
  Ttb_max : Saturate  UpperLimit=Ttb_max  LowerLimit=-Ttb_max
  xtd(t) : Outport
  dxtd(t) : Outport  Port=2
  theta_tm(t) : Outport  Port=3
  wires:
  Integrator1/1 -> xtd(t)/1
  Sum/1 -> Gain/1
  Integrator/1 -> Integrator1/1, Gain4/1, dxtd(t)/1, Gain1/1  "dxtd(t)"
  Ftw(t)/1 -> Sum/1
  Gain2/1 -> Sum/2
  Gain1/1 -> Sum/3
  Gain/1 -> Integrator/1  "ddxtd(t)"
  Ttm/1 -> Sum1/1
  Sum1/1 -> Gain2/1
  Product/1 -> Ttb_max/1
  Ttb/1 -> Product/1  "OpBrake Control Signal"
  Ttb_max/1 -> Sum1/2
  Gain3/1 -> Product/2
  Gain4/1 -> Gain5/1  "wtd(t)"
  Gain5/1 -> Integrator2/1, Gain3/1  "wtm(t)"
  Integrator2/1 -> theta_tm(t)/1

== system Plant/Trolley Drive/Trolley Cable Mode ==
  note: Trolley Cable Mode (Eq 4.a)
  xt(t) : Inport
  dxt(t) : Inport  Port=2
  xtd(t) : Inport  Port=3
  dxtd(t) : Inport  Port=4
  Gain : Gain  Gain=Ktw
  Gain1 : Gain  Gain=btw
  Sum : Sum  Inputs=+|+
  Sum1 : Sum  Inputs=|+-
  Sum3 : Sum  Inputs=|+-
  Ftw : Outport
  wires:
  Sum/1 -> Ftw/1
  xtd(t)/1 -> Sum1/1
  xt(t)/1 -> Sum1/2
  Sum1/1 -> Gain/1
  Gain/1 -> Sum/1
  Gain1/1 -> Sum/2
  Sum3/1 -> Gain1/1
  dxtd(t)/1 -> Sum3/1
  dxt(t)/1 -> Sum3/2

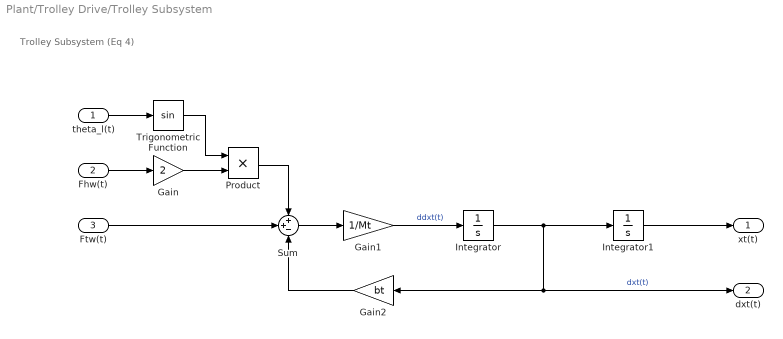
== system Plant/Trolley Drive/Trolley Subsystem ==
  note: Trolley Subsystem (Eq 4)
  theta_l(t) : Inport
  Fhw(t) : Inport  Port=2
  Ftw(t) : Inport  Port=3
  Gain : Gain  Gain=2
  Gain1 : Gain  Gain=1/Mt
  Gain2 : Gain  Gain=bt
  Integrator : Integrator  InitialCondition=dxt0
  Integrator1 : Integrator  InitialCondition=xt0
  Product : Product
  Sum : Sum  Inputs=++-
  Trigonometric Function : Trigonometry
  xt(t) : Outport
  dxt(t) : Outport  Port=2
  wires:
  Ftw(t)/1 -> Sum/2
  Trigonometric Function/1 -> Product/1
  Gain1/1 -> Integrator/1  "ddxt(t)"
  Sum/1 -> Gain1/1
  Integrator/1 -> Integrator1/1, Gain2/1, dxt(t)/1  "dxt(t)"
  Product/1 -> Sum/1
  theta_l(t)/1 -> Trigonometric Function/1
  Integrator1/1 -> xt(t)/1
  Fhw(t)/1 -> Gain/1
  Gain/1 -> Product/2
  Gain2/1 -> Sum/3

== stateflow chart Plant/Animation/Chart ==
  state MAIN [parallel]
    settings: executionOrder=1
    state Loose
    state Latched
      during:
      X=XS;
      Y=YS-1.2;
    (default) -> Loose : {X=X0;
        | Y=Y0;}
    Loose -> Latched : [Latch==1]
    Latched -> Loose : [Latch==0]
  state LacthEvaluator [parallel]
    Latch=0;
    TLK_1=0;
    during:
    if abs(XS-X)<0.2 && abs(YS-Y)<0.2 && TLK~=TLK_1 && Latch==0
    Latch=1;
    end
    if Latch==1 && TLK~=TLK_1
    Latch=0;
    end
    TLK_1=TLK;
    settings: executionOrder=2
  data: Y output; X output; TLK_1 local; Latch local; XS input; YS input; TLK input; Y0 input; X0 input

== stateflow chart Plant/Container Profile/Container Profile Manager ==
  state Start
    entry:
    layout = containerLayout;
    masses = containerMasses;
  state On
    during:
    index = floor(xl/Hc)+1;
    if index > length(layout)
    c = -1;
    else
    c = layout(index);
    end
    yc0 = get_yc0(layout, xl, Hc);
    note: should only be able to take the container if the spreader is over it and distance yl - yc0 is close to zero
    state PickUpContainer
      entry:
      layout(index) = c-1;
      Mc = masses(index);
      m = randi([massRange(1), massRange(2)]);
      masses(index) = m;
    state LayoutUnchanged
    state DropContainer
      entry:
      layout(index) = c+1;
      Mc = 0;
      m = randi([massRange(1), massRange(2)]);
      masses(index) = m;
    (default) -> LayoutUnchanged
    PickUpContainer -> LayoutUnchanged : [TLK_up == 0]
    LayoutUnchanged -> PickUpContainer [order 1] : [TLK_up == 1]
    LayoutUnchanged -> DropContainer [order 2] : [TLK_down == 1]
    DropContainer -> LayoutUnchanged : [TLK_down == 0]
  (default) -> Start
  Start -> On
  data: Layout function_input; x_query function_input; containerWidth_ function_input; profileHeight function_output; containerLayout input; xl input; TLK_up input; yc0 output; Hc input; c local; index local; TLK_down input; layout output; containerMasses input; masses local; Mc output; massRange input; m local
  function profileHeight = get_yc0(Layout, x_query, containerWidth_):
    | function profileHeight = get_yc0(Layout, x_query, containerWidth_)
    | %% CONTAINER PROFILE -- constant container height = 2.5m
    |     cols = length(Layout);
    |     Nc = containerWidth_/0.1;
    |     
    |     containerProfile=zeros(1,cols*Nc);
    |     
    |     for i=1:cols
    |         for j=1:Nc
    |             stackHeight = 0;%Layout(i)*containerHeight;
    |             if i==1 && j==1 %first iteration
    |                 containerProfile = stackHeight;
    |             else
    |                 containerProfile = [containerProfile, stackHeight];
    |             end
    |         end
    |     end
    | 
    | 
    | %% GENERATE FULL OBSTACLE PROFILE
    |     containerWidth_ = 2.5;
    |     xmin = -30;
    |     xmax = 50;
    |     dx = 0.1;
    |     N = (xmax - xmin)/dx + 1;
    |     Ob_profile = zeros(N,2);
    |     Ob_profile(:,1) = (xmin:0.1:xmax)';
    |     
    |     % Loading Bay1 - Bahia de carga 
    |     Ob_profile=ObstUpdate(Ob_profile,-23.5,-20.5,1);
    |     
    |     % Loading Bay2 - Bahia de carga 
    |     Ob_profile=ObstUpdate(Ob_profile,-16.5,-13.5,1);
    |     
    |     % Loading Bay3 - Bahia de carga 
    |     Ob_profile=ObstUpdate(Ob_profile,-9.5,-7.5,1);
    |     
    |     % Sill Beam - Viga Grua
    |     Ob_profile=ObstUpdate(Ob_profile,-2,0,15);
    |     
    |     % Gap 
    |     Ob_profile=ObstUpdate(Ob_profile,0,0.5,-2);
    |     
    |     % Ship wall - Pared barco
    |     Ob_profile=ObstUpdate(Ob_profile,0.5,1.5,5);
    |     
    |     % Ship floor - Piso barco
    |     Ob_profile=ObstUpdate(Ob_profile,1.5,24.9,-19);
    |     
    |     % Ship wall - Pared barco
    |     Ob_profile=ObstUpdate(Ob_profile,24.9,25.9,5);
    |     
    |     
    | %% Get yc0 at x_query
    |     y1 = interp1(Ob_profile(:,1), Ob_profile(:,2), x_query, 'previous');
    |     y2 = interp1(Ob_profile(:,1), Ob_profile(:,2), x_query, 'next');
    |     profileHeight = max(y1, y2);
    | 
    | 
    | end
    | 
    | 
    | function NewProfile=ObstUpdate(OldProfile,x0,x1,y)
    | NewProfile=OldProfile;
    | i=1;
    | while NewProfile(i,1)<x0
    |     i=i+1;
    | end
    | while NewProfile(i,1)<x1
    |     i=i+1;
    |     NewProfile(i,2)=y;
    | end
    | end
